simulink model "SimulaPID"  (R2018a)
settings: Solver=VariableStepAuto  StartTime=0.0  StopTime=250  RelTol=1e-3
values from neighbouring files (symbols this model uses):
  Kc = (1/(2*L))*(1/(Ke/Ti))    (= 0.102221616464)    [Analise_robustez_q4.m]    (also in psfRapido.m; psfRapido_IMC.m; scriptAux.m)
  Td = t2    (= 0.2)    [Analise_robustez_q4.m]    (also in psfRapido.m; psfRapido_IMC.m; scriptAux.m)
  Ti = t1    (= 0.45)    [Analise_robustez_q4.m]    (also in psfRapido.m; psfRapido_IMC.m; scriptAux.m)
libraries: simulink x4
settings Model: Creator=julia  LastModifiedBy=crist
settings CodeAppCC: StateflowObjectComments=on

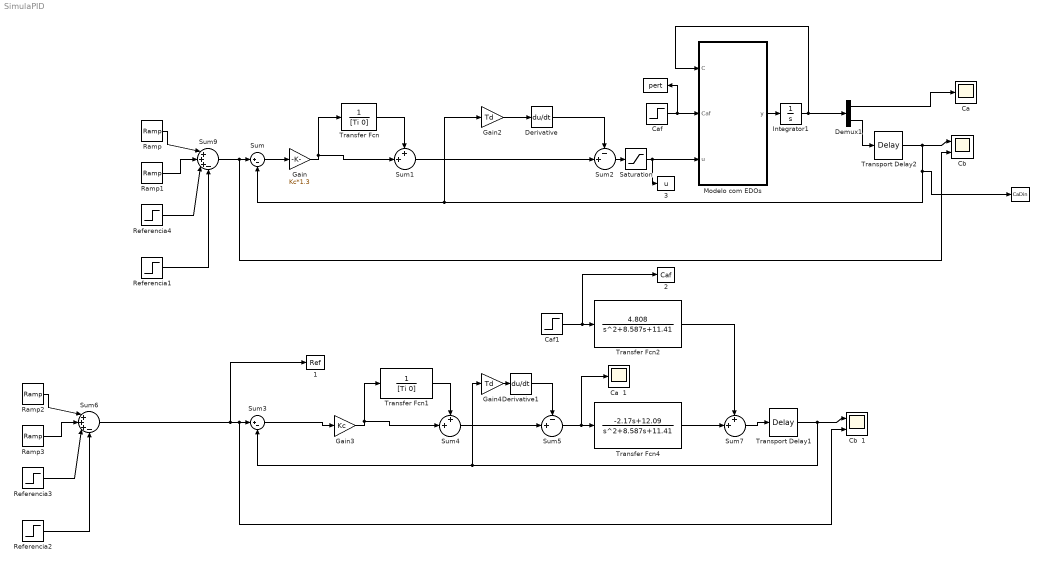
== system SimulaPID ==
  "          " : ToWorkspace  VariableName=pert  SaveFormat=Timeseries  SampleTime=-1
  "                   " : ToWorkspace  VariableName=CaDin  SaveFormat=Timeseries  SampleTime=-1
  "                   1" : ToWorkspace  VariableName=Ref  SaveFormat=Timeseries  SampleTime=-1
  "                   2" : ToWorkspace  VariableName=Caf  SaveFormat=Timeseries  SampleTime=-1
  "                   3" : ToWorkspace  VariableName=u  SaveFormat=Timeseries  SampleTime=-1
  "Ca  " : Scope
  Ca  1 : Scope
  Caf : Step  Time=180  Before=5.1  After=5.2  SampleTime=0
  Caf1 : Step  Time=180  After=0.1  SampleTime=0
  "Cb  " : Scope  NumInputPorts=2
  Cb  1 : Scope  NumInputPorts=2
  Demux1 : Demux  Outputs=2
  Derivative : Derivative
  Derivative1 : Derivative
  Gain : Gain  Gain=Kc*1.3
  Gain2 : Gain  Gain=Td
  Gain3 : Gain  Gain=Kc
  Gain4 : Gain  Gain=Td
  Integrator1 : Integrator  InitialCondition=[0;0]
  Modelo com EDOs : MATLAB Function  TreatAsAtomicUnit=on
  Ramp : simulink/Sources/Ramp  slope=2.345/50  start=0  InitialOutput=0
  Ramp1 : simulink/Sources/Ramp  slope=-2.345/50  start=50  InitialOutput=0
  Ramp2 : simulink/Sources/Ramp  slope=2.345/50  start=0  InitialOutput=0
  Ramp3 : simulink/Sources/Ramp  slope=-2.345/50  start=50  InitialOutput=0
  Referencia1 : Step  Time=140  After=0  SampleTime=0
  Referencia2 : Step  Time=140  After=0  SampleTime=0
  Referencia3 : Step  Time=130  After=0.25  SampleTime=0
  Referencia4 : Step  Time=130  After=0.25  SampleTime=0
  Saturation : Saturate  UpperLimit=5  LowerLimit=0
  Sum : Sum  Inputs=|+-
  Sum1 : Sum  Inputs=++|
  Sum2 : Sum  Inputs=-+|
  Sum3 : Sum  Inputs=|+-
  Sum4 : Sum  Inputs=++|
  Sum5 : Sum  Inputs=-+|
  Sum6 : Sum  Inputs=|+++-
  Sum7 : Sum  Inputs=++|
  Sum9 : Sum  Inputs=|+++-
  Transfer Fcn : TransferFcn  Denominator=[Ti 0]
  Transfer Fcn1 : TransferFcn  Denominator=[Ti 0]
  Transfer Fcn2 : TransferFcn  Numerator=[4.808]  Denominator=[1 8.587 11.41]
  Transfer Fcn4 : TransferFcn  Numerator=[-2.17 12.09]  Denominator=[1 8.587 11.41]
  Transport Delay1 : TransportDelay  DelayTime=3
  Transport Delay2 : TransportDelay  DelayTime=3
  wires:
  Modelo com EDOs/1(y) -> Integrator1/1
  Integrator1/1 -> Modelo com EDOs/1(C), Demux1/1
  Demux1/1 -> "Ca  "/1
  Caf/1 -> "          "/1, Modelo com EDOs/2(Caf)
  Referencia4/1 -> Sum9/3
  Sum9/1 -> Sum/1, "Cb  "/2
  Ramp1/1 -> Sum9/2
  Ramp/1 -> Sum9/1
  Demux1/2 -> Transport Delay2/1
  Transport Delay2/1 -> "                   "/1, Sum/2, Gain2/1, "Cb  "/1
  Gain/1 -> Sum1/2, Transfer Fcn/1
  Transfer Fcn/1 -> Sum1/1
  Sum1/1 -> Sum2/2
  Sum/1 -> Gain/1
  Referencia1/1 -> Sum9/4
  Gain2/1 -> Derivative/1
  Sum5/1 -> Ca  1/1, Transfer Fcn4/1
  Gain3/1 -> Sum4/2, Transfer Fcn1/1
  Transfer Fcn1/1 -> Sum4/1
  Transport Delay1/1 -> Gain4/1, Sum3/2, Cb  1/1
  Sum4/1 -> Sum5/2
  Sum3/1 -> Gain3/1
  Gain4/1 -> Derivative1/1
  Derivative1/1 -> Sum5/1
  Referencia3/1 -> Sum6/3
  Ramp3/1 -> Sum6/2
  Ramp2/1 -> Sum6/1
  Referencia2/1 -> Sum6/4
  Transfer Fcn4/1 -> Sum7/2
  Sum7/1 -> Transport Delay1/1
  Transfer Fcn2/1 -> Sum7/1
  Caf1/1 -> "                   2"/1, Transfer Fcn2/1
  Sum6/1 -> "                   1"/1, Sum3/1, Cb  1/2
  Derivative/1 -> Sum2/1
  Sum2/1 -> Saturation/1
  Saturation/1 -> Modelo com EDOs/3(u), "                   3"/1

== matlab function SimulaPID/Modelo com EDOs ==
  data: y output; C input; Caf input; u input
%EDOs das concentracoes dos produtos A e B
function y = fcn(C, Caf, u)

%constantes
k1 = 6.01; %L/min
k2 = 0.8433; %L/min
k3 = 0.1123; %mol/Lmin

%variaveis das concentracoes dos produtos A e B
Ca = C(1);
Cb = C(2);

%EDOs
Ca_d = -k1*Ca - k3*(Ca^2) + (Caf - Ca)*u;
Cb_d =  k1*Ca - k2*Cb - Cb*u;
 
%conjunto das EDOs
y = [Ca_d;Cb_d];
